simulink library "LibControllers"  (R2015b)
settings: Solver=ode45  SolverMode=SingleTasking  StartTime=0.0  StopTime=10.0  RelTol=1e-3
undefined symbols (not defined in the file or in its folder): accelCanon, adjustCoefficients, bw, depth, DiscIntNeverNeededParam, displCanon, forget, freq, initDispl, jerkCanon, kd, kdp, kf, ki, kp, maxAuthority, maxForce, nominFlow, p, R, ratedFlow, S, samplePeriod, T, velocCanon
undefined symbols (not defined in the file): fbkgen, fdp, fmax, fmin, gainRatio, interval, lagFreq, lagPhase, leadFreq, leadPhase, order, refabort, refgen, refsmooth, supplyPress, vmax, vmin
libraries: LibControllers x43, simulink x1
(part 1 of 2)
settings Model: Creator=THOENB  LastModifiedBy=Andreas
settings DataIOCC: SaveFormat=Array  SignalLoggingSaveFormat=ModelDataLogs
settings OptimizationCC: BlockReduction=off  BooleanDataType=off  ExpressionDepthLimit=2147483647
settings DebuggingCC: SaveWithParameterizedLinksMsg=none  UnderspecifiedInitializationDetection=Classic  MergeDetectMultiDrivingBlocksExec=none  SignalResolutionControl=TryResolveAllWithWarning  FcnCallInpInsideContextMsg=UseLocalSettings  StateNameClashWarn=warning  StrictBusMsg=Warning
settings HardwareCC: ProdBitPerPointer=32  ProdLargestAtomicFloat=None  ProdIntDivRoundTo=Undefined  ProdEndianess=Unspecified  ProdWordSize=32  ProdHWDeviceType=32-bit Generic  TargetUnknown=on
settings GRTTargetCC: GeneratePreprocessorConditionals=Disable all  CombineOutputUpdateFcns=off  GRTInterface=on
settings ConfigComp: CovModelRefEnable=Off

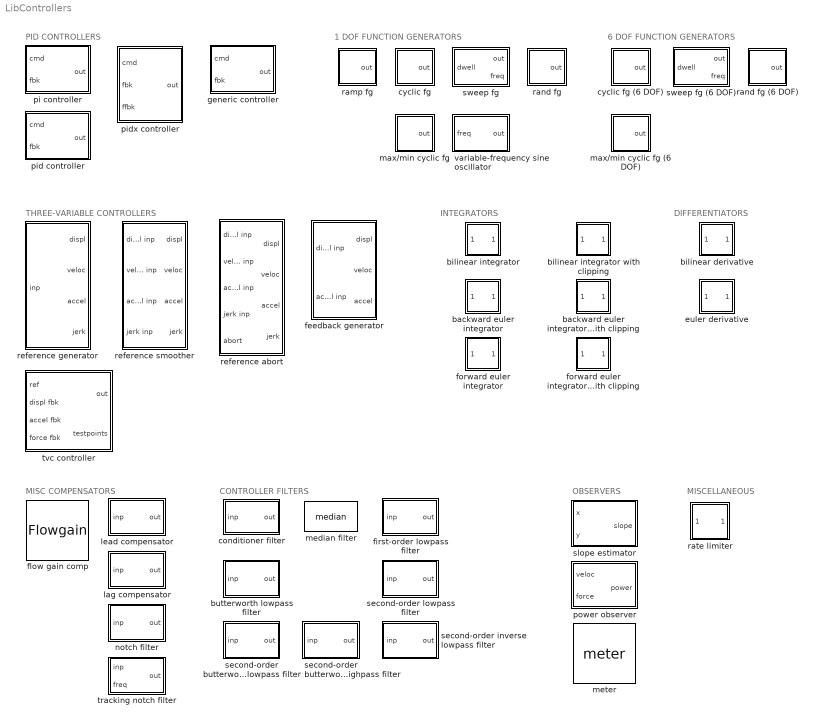
== system LibControllers ==
  note: PID CONTROLLERS
  note: MISC COMPENSATORS
  note: THREE-VARIABLE CONTROLLERS
  note: CONTROLLER FILTERS
  note: OBSERVERS
  note: 1 DOF FUNCTION GENERATORS
  note: INTEGRATORS
  note: DIFFERENTIATORS
  note: 6 DOF FUNCTION GENERATORS
  note: MISCELLANEOUS
  backward euler integrator : Subsystem  mask(Discrete Backward Euler Integrator){initialCondition=0, samplePeriod=samplePeriod}
      mask prompts: initialCondition "Initial condition"; samplePeriod "Sample period (sec)"
      mask Display: dpoly('[T]', [1 -1], 'z-')
  backward euler integrator with clipping : Subsystem  mask(Discrete Backward Euler Integrator with Clipping){initialCondition=0, maxOutput=inf, minOutput=-inf, samplePeriod=samplePeriod}
      mask prompts: initialCondition "Initial condition"; maxOutput "Maximum output"; minOutput "Minimum output"; samplePeriod "Sample period (sec)"
      mask Display: dpoly('[T]', [1 -1], 'z-')
  bilinear derivative : Subsystem  mask(Discrete Bilinear Differentiator){decay=0.9, initialCondition=0, samplePeriod=samplePeriod}
      mask prompts: decay "Decay time constant (0: backward Euler, 1: binlinear)"; initialCondition "Initial condition"; samplePeriod "Sample period"
      mask Display:
      | text(0.1,.75,'2');
      | text(0.1,.65,'_');
      | text(0.1,.25,'T');
      | text(.3,.80,'{1-z}^{-1}', 'hor','left','texmode','on');
      | text(.3,.65,'___');
      | text(.3,.30,'{1+z}^{-1}', 'hor','left','texmode','on');
  bilinear integrator : Subsystem  mask(Discrete Bilinear Integrator){initialCondition=0, samplePeriod=samplePeriod}
      mask prompts: initialCondition "Initial condition"; samplePeriod "Sample period (sec)"
      mask Display:
      | text(0.1,.75,'T');
      | text(0.1,.65,'_');
      | text(0.1,.25,'2');
      | text(.3,.80,'{1+z}^{-1}', 'hor','left','texmode','on');
      | text(.3,.65,'___');
      | text(.3,.30,'{1-z}^{-1}', 'hor','left','texmode','on');
  bilinear integrator with clipping : Subsystem  mask(Discrete Bilinear Integrator with Clipping){initialCondition=0, maxOutput=inf, minOutput=-inf, samplePeriod=samplePeriod}
      mask prompts: initialCondition "Initial condition"; maxOutput "Maximum output"; minOutput "Minimum output"; samplePeriod "Sample period (sec)"
      mask Display:
      | text(0.1,.75,'T');
      | text(0.1,.65,'_');
      | text(0.1,.25,'2');
      | text(.3,.80,'{1+z}^{-1}', 'hor','left','texmode','on');
      | text(.3,.65,'___');
      | text(.3,.30,'{1-z}^{-1}', 'hor','left','texmode','on');
  butterworth lowpass filter : Subsystem  mask(Butterworth Lowpass Filter){freq=bw, n=order, samplePeriod=samplePeriod}
      mask prompts: freq "Bandwidth (Hz)"; n "Filter order"; samplePeriod "Sample period (sec)"
      mask init:
      | fsamp = 1 / samplePeriod;
      | maxNSos	= 15;	% define maximum number of second-order sections
      | if (0 < freq) && (freq < 0.5 * fsamp) && (0 < n)
      | 	wn = freq / (0.5 * fsamp);
      | 	[z, p, k] = butter(n, wn, 'low');
      | else
      | 	[z, p, k] = tf2zpk([1], [1]);
      | end
      | [sos, g] = zp2sos(z, p, k);	% convert to second-order sections
      | 
      | % fix passband gain bug in cheby1()
      | % (note:  can't use freqz() for a single frequency)
      | wn = 0;
      | zexp = [1 exp(-1*j*wn) exp(-2*j*wn)]';
      | h = 1;
      | for i = 1:size(sos,1)
      | 	b = sos(i, 1:3);
      | 	a = sos(i, 4:6);
      | 	h = h * (b * zexp) / (a * zexp);
      | end
      | g = 1 / abs(h);
      | 
      | % check filter length
      | nSos = size(sos,1);
      | if nSos > maxNSos
      | 	fstr = ['Max number of second-order filter sections' ...
      | 			' (%u) exceeded: %u'];
      | 	error(sprintf(fstr, maxNSos, nSos));
      | end
      | 
      | % pad number of second-order filter sections up to the maximum
      | sos = [sos; repmat([1 0 0 1 0 0], maxNSos-nSos, 1)];
  conditioner filter : Subsystem  mask(Conditioner Filter){filterType=Elliptic, freq3dB=freq, samplePeriod=samplePeriod}
      mask prompts: filterType "Filter type"; freq3dB "3 dB cutoff frequency (inf, 1000, 500, 300, 100, 50 Hz)"; samplePeriod "Sample period (sec)"
      mask init:
      | fsamp = 1 / samplePeriod;
      | switch filterType
      | 	case 1	% bessel
      | 		% note:  higher 3dB frequency mapping 
      | 		% is accurate only for fsamp = 2048
      | 		if isempty(freq3dB)
      | 			freq3dB = fsamp;
      | 		elseif freq3dB == 1000
      | 			freq3dB = fsamp;
      | 		elseif freq3dB == 500
      | 			freq3dB = 1018.9;
      | 		elseif freq3dB == 300
      | 			freq3dB = 524.0;
      | 		elseif freq3dB == 100
      | 			freq3dB = 163.4;
      | 		elseif freq3dB == 50
      | 			freq3dB = 81.23;
      | 		else
      | 			freq3dB = fsamp;
      | 		end
      | 		if freq3dB > fsamp/2
      | 			a = [1];
      | 			b = [1];
      | 		else
      | 			[b, a] = besself(5, 2*pi*freq3dB);
      | 			[b, a] = bilinear(b, a, fsamp);
      | 		end
      | 	case 2	% butterworth
      | 		if freq3dB > fsamp/2
      | 			a = [1];
      | 			b = [1];
      | 		else
      | 			[b, a] = butter(5, 2*freq3dB/fsamp);
      | 		end
      | 	case 3	% elliptic
      | 		% note:  higher 3dB frequency mapping 
      | 		% is accurate only for fsamp = 2048
      | 		if isempty(freq3dB)
      | 			freq3dB = fsamp;
      | 		elseif freq3dB == 1000
      | 			freq3dB = 980.6;
      | 		elseif freq3dB == 500
      | 			freq3dB = 319.3;
      | 		elseif freq3dB == 300
      | 			freq3dB = 174.4;
      | 		elseif freq3dB == 100
      | 			freq3dB = 55.60;
      | 		elseif freq3dB == 50
      | 			freq3dB = 27.69;
      | 		else
      | 			freq3dB = fsamp;
      | 		end
      | 		if freq3dB > fsamp/2
      | 			a = [1];
      | 			b = [1];
      | 		else
      | 			[b, a] = ellip(4, 0.001, 60.0, 2*freq3dB/fsamp);
      | 		end
      | end
      mask TypeOptions filterType: Bessel | Butterworth | Elliptic
  cyclic fg : Subsystem  mask(Cyclic Function Generator){shape=Sine, ampl=1, freq=1, phase=0, spanInterval=1, samplePeriod=samplePeriod, triggered=off}
      mask prompts: ampl "Amplitude"; freq "Frequency (Hz)"; phase "Phase (deg)"; spanInterval "Span interval (sec)"; samplePeriod "Sample period (sec)"; triggered "Used in Triggered Subsystem"
      mask init:
      | if triggered
      | 	sourceSamplePeriod = -1;
      | else
      | 	sourceSamplePeriod = samplePeriod;
      | end
      | freq = max(freq, eps);
      mask TypeOptions shape: Square | Triangle | Sine
  cyclic fg (6 DOF) : Subsystem  mask(Cyclic Function Generator (6 DOF)){id=x, shape=Sine, ampl=1, freq=1, phase=0, spanInterval=1, samplePeriod=samplePeriod, dof=1:6, triggered=off}
      mask prompts: id "DOF"; ampl "Amplitude"; freq "Frequency (Hz)"; phase "Phase (deg)"; spanInterval "Span interval (sec)"; samplePeriod "Sample period (sec)"; dof "Degree-of-freedom indices (1: X; 2: Y; 3: Z; 4: Roll; 5: Pitch; 6: Yaw)"; triggered "Used in Triggered Subsystem"
      mask init:
      | if triggered
      | 	sourceSamplePeriod = -1;
      | else
      | 	sourceSamplePeriod = samplePeriod;
      | end
      mask TypeOptions id: x | y | z | roll | pitch | yaw
      mask TypeOptions shape: Square | Triangle | Sine
  euler derivative : Subsystem  mask(Discrete Euler Derivative){initialCondition=0, samplePeriod=samplePeriod}
      mask prompts: initialCondition "Initial condition"; samplePeriod "Sample period (sec)"
      mask Display: dpoly([1 -1], '[T]', 'z-')
  feedback generator : Subsystem  mask(Feedback Generator){freq=fbkgen.freq, damp=fbkgen.damp, direct=fbkgen.direct, displCanon=displCanon, velocCanon=velocCanon, accelCanon=accelCanon, initDispl=initDispl, samplePeriod=samplePeriod}
      mask prompts: freq "Crossover frequency (Hz)"; damp "Damping ratio"; direct "Direct displacement (0: indirect, 1: direct)"; displCanon "Canonical displacement units"; velocCanon "Canonical velocity units"; accelCanon "Canonical acceleration units"; initDispl "Initial displacement"; samplePeriod "Sample period (sec)"
      mask init:
      | omega = 2 * pi * freq;
      | a0    = omega * omega * omega;
      | a1    = (2 * damp + 1) * omega * omega;
      | a2    = (2 * damp + 1) * omega;
  first-order lowpass filter : Subsystem  mask(First-Order Lowpass Filter){freq=100, samplePeriod=samplePeriod}
      mask prompts: freq "Frequency (Hz)"; samplePeriod "Sample period (sec)"
      mask init:
      | fsamp = 1 / samplePeriod;
      | if ((0 < freq) && (freq < 0.5 * fsamp))
      | 	bwt	= freq * samplePeriod;
      | 	c	= 1.0 / tan(pi * bwt);	% prewarp
      | 	bwt	= 1.0 / (pi * c);
      | 	a0	= 1.0;
      | 	a1	= -exp(-2 * pi * bwt);
      | 	b0	= 1 + a1;
      | 	b1	= 0;
      | 	a	= [a0 a1];
      | 	b	= [b0 b1];
      | else
      | 	a = [1];
      | 	b = [1];
      | end
  flow gain comp : S-Function  FunctionName=Flowgain  Parameters=[satAuth droopAuth switchAuth ratedFlow nominFlow nomPress minPress maxForce]  SFunctionDeploymentMode=off  EnableBusSupport=off  mask(Flow Gain Compensator){satAuth=1, droopAuth=1, switchAuth=1, ratedFlow=ratedFlow, nominFlow=nominFlow, nomPress=supplyPress, minPress=supplyPress/3, maxForce=maxForce}
      mask prompts: satAuth "Valve saturation authority"; droopAuth "Supply pressure droop authority"; switchAuth "Pressure switching authority"; ratedFlow "Rated flow"; nominFlow "Nominal flow"; nomPress "Nominal supply pressure"; minPress "Minimum supply pressure"; maxForce "Maximum force at nominal supply pressure"
      mask Display:
      | disp('');
      | port_label('input', 1, 'inp');
      | port_label('input', 2, 'press');
      | port_label('input', 3, 'force');
      | port_label('output', 1, 'out');
      | port_label('output', 2, 'gain');
  forward euler integrator : Subsystem  mask(Discrete Forward Euler Integrator){initialCondition=0, samplePeriod=samplePeriod}
      mask prompts: initialCondition "Initial condition"; samplePeriod "Sample period (sec)"
      mask Display:
      | text(.25,.80,'{Tz}^{-1}', 'hor','left','texmode','on');
      | text(.25,.65,'___');
      | text(.25,.30,'{1-z}^{-1}', 'hor','left','texmode','on');
  forward euler integrator with clipping : Subsystem  mask(Discrete Forward Euler Integrator with Clipping){initialCondition=0, maxOutput=inf, minOutput=-inf, samplePeriod=samplePeriod}
      mask prompts: initialCondition "Initial condition"; maxOutput "Maximum output"; minOutput "Minimum output"; samplePeriod "Sample period (sec)"
      mask Display:
      | text(.25,.80,'{Tz}^{-1}', 'hor','left','texmode','on');
      | text(.25,.65,'___');
      | text(.25,.30,'{1-z}^{-1}', 'hor','left','texmode','on');
  generic controller : Subsystem  mask(Generic Controller){R=R, S=S, T=T, k=1}
      mask prompts: R "Regression polynomial"; S "Feedback polynomial"; T "Feedforward polynomial"; k "Output scaling"
  lag compensator : Subsystem  mask(Lag compensator){lagPhase=lagPhase, lagFreq=lagFreq, gainRatio=gainRatio, samplePeriod=samplePeriod}
      mask prompts: lagPhase "Lag phase ([]: use minimum possible) (deg)"; lagFreq "Lag frequency (Hz)"; gainRatio "Gain ratio (high frequency attenuation)"; samplePeriod "Sample period (sec)"
      mask init:
      | fsamp = 1 / samplePeriod;
      | if isempty(lagPhase)
      | 	lagPhase = 0;
      | end
      | 
      | % return wire if attenuation or lag frequency is zero
      | a = [1];
      | b = [1];
      | if ~(gainRatio > 0) || ~(lagFreq > 0)
      |     return
      | end
      | k         = 1 / gainRatio;
      | lagPhase  = -abs(lagPhase);
      |  
      | % determine compensator damping
      | centOmega = 2*pi*lagFreq;
      | phi       = (lagPhase / 2) * pi/180;
      | maxPhase  = 89.0 * pi/180;
      | phi       = min(phi, maxPhase);
      | tanphi    = tan(phi);
      | damp      = ((sqrt(k)-1))/(2*sqrt(sqrt(k))) / tanphi;
      |  
      | % design laplace domain compensator
      | zeroOmega = centOmega / sqrt(sqrt(k));
      | poleOmega = centOmega * sqrt(sqrt(k));
      | scale     = (poleOmega / zeroOmega)^2;
      | a         = [1 2*damp*poleOmega poleOmega^2];
      | b         = [1 2*damp*zeroOmega zeroOmega^2] * scale;
      |  
      | % transform to z domain using bilinear transformation with prewarping
      | if ~isempty(fsamp) && (lagPhase < 0)
      | 	omega = centOmega;
      | 	as   = a;
      | 	bs   = b;
      | 	a    = zeros(1, 3);
      | 	b    = zeros(1, 3);
      | 	c    = omega / tan(omega / (2*fsamp));
      | 	cc   = c * c;
      | 	d    = as(3) + as(2)*c + as(1)*cc;
      | 	a(1) = 1.0;
      | 	a(2) =  2.0*(as(3)-as(1)*cc)/d;
      | 	a(3) = (as(3)-as(2)*c+as(1)*cc)/d;
      | 	b(1) = (bs(3)+bs(2)*c+bs(1)*cc)/d;
      | 	b(2) =  2.0*(bs(3)-bs(1)*cc)/d;
      | 	b(3) = (bs(3)-bs(2)*c+bs(1)*cc)/d;
      | end
  lead compensator : Subsystem  mask(Lead compensator){leadPhase=leadPhase, leadFreq=leadFreq, gainRatio=gainRatio, samplePeriod=samplePeriod}
      mask prompts: leadPhase "Lead phase (deg)"; leadFreq "Lead frequency (Hz)"; gainRatio "Gain ratio ([]: use maximum possible)"; samplePeriod "Sample period (sec)"
      mask init:
      | fsamp = 1 / samplePeriod;
      | if isempty(gainRatio)
      | 	gainRatio = Inf;
      | end
      | 
      | % return wire if lead phase or lead frequency is zero
      | a = [1];
      | b = [1];
      | if ~(leadPhase > 0) || ~(leadFreq > 0)
      |     return
      | end
      | leadPhase = leadPhase * pi/180;
      | maxPhase  = 89.0 * pi/180;
      | 
      | % limit gain ratio
      | minGainRatio = 1.001;
      | maxGainRatio = 1000;
      | k            = min(max(gainRatio, minGainRatio), maxGainRatio);
      |  
      | % determine compensator damping
      | centOmega = 2*pi*leadFreq;
      | phi       = leadPhase / 2;
      | phi       = min(phi, maxPhase);
      | tanphi    = tan(phi);
      | damp      = ((sqrt(k) - 1) / (2*sqrt(sqrt(k)))) / tanphi;
      | damp      = min(damp, 1);
      | k         = (damp*tanphi + sqrt((damp*tanphi)^2 + 1))^4;
      |  
      | % design laplace domain compensator
      | zeroOmega = centOmega / sqrt(sqrt(k));
      | poleOmega = centOmega * sqrt(sqrt(k));
      | scale     = sqrt( (  (poleOmega^2-centOmega^2)^2 ...
      |                    + (2*damp*poleOmega*centOmega)^2) ...
      |                  / ( (zeroOmega^2-centOmega^2)^2 ...
      |                     + (2*damp*zeroOmega*centOmega)^2));
      | a         = [1 2*damp*poleOmega poleOmega^2];
      | b         = [1 2*damp*zeroOmega zeroOmega^2] * scale;
      |  
      | % transform to z domain using bilinear transformation with prewarping
      | if ~isempty(fsamp) && (leadPhase > 0)
      | 	omega = centOmega;
      | 	as   = a;
      | 	bs   = b;
      | 	a    = zeros(1, 3);
      | 	b    = zeros(1, 3);
      | 	c    = omega / tan(omega / (2*fsamp));
      | 	cc   = c * c;
      | 	d    = as(3) + as(2)*c + as(1)*cc;
      | 	a(1) = 1.0;
      | 	a(2) =  2.0*(as(3)-as(1)*cc)/d;
      | 	a(3) = (as(3)-as(2)*c+as(1)*cc)/d;
      | 	b(1) = (bs(3)+bs(2)*c+bs(1)*cc)/d;
      | 	b(2) =  2.0*(bs(3)-bs(1)*cc)/d;
      | 	b(3) = (bs(3)-bs(2)*c+bs(1)*cc)/d;
      | end
  max/min cyclic fg : Subsystem  mask(Max/Min Cyclic Function Generator){shape=Triangle, startLevel=0, endLevel=1, freq=1, samplePeriod=samplePeriod, triggered=off}
      mask prompts: startLevel "Starting level"; endLevel "Ending level"; freq "Frequency (Hz)"; samplePeriod "Sample period (sec)"; triggered "Used in Triggered Subsystem"
      mask init:
      | mean  = (startLevel + endLevel) / 2;
      | ampl  = (startLevel - endLevel) / 2;
      | phase = sign(ampl) * 90;
      | ampl  = abs(ampl);
      | if shape == 1	% square
      | 	phase = phase - 90;
      | end
      | if triggered
      | 	sourceSamplePeriod = -1;
      | else
      | 	sourceSamplePeriod = samplePeriod;
      | end
      | freq = max(freq, eps);
      mask TypeOptions shape: Square | Triangle | Sine
  max/min cyclic fg (6 DOF) : Subsystem  mask(Max/Min Cyclic Function Generator (6 DOF)){id=x, shape=Sine, startLevel=0, endLevel=1, freq=1, samplePeriod=samplePeriod, dof=1:6, triggered=off}
      mask prompts: id "DOF"; startLevel "Starting level"; endLevel "Ending level"; freq "Frequency (Hz)"; samplePeriod "Sample period (sec)"; dof "Degree-of-freedom indices (1: X; 2: Y; 3: Z; 4: Roll; 5: Pitch; 6: Yaw)"; triggered "Used in Triggered Subsystem"
      mask init:
      | mean  = (startLevel + endLevel) / 2;
      | ampl  = (startLevel - endLevel) / 2;
      | phase = sign(ampl) * 90;
      | ampl  = abs(ampl);
      | if shape == 1	% square
      | 	phase = phase - 90;
      | end
      | if triggered
      | 	sourceSamplePeriod = -1;
      | else
      | 	sourceSamplePeriod = samplePeriod;
      | end
      mask TypeOptions id: x | y | z | roll | pitch | yaw
      mask TypeOptions shape: Square | Triangle | Sine
  median filter : S-Function  FunctionName=median  Parameters=width  SFunctionDeploymentMode=off  EnableBusSupport=off  mask(Median filter){width=1}
      mask prompts: width "Glitch width (samples)"
  meter : S-Function  FunctionName=meter  Parameters=[mode band decay samplePeriod]  SFunctionDeploymentMode=off  EnableBusSupport=off  mask(Signal Meter){mode=max/min, band=0.1, decay=1, samplePeriod=samplePeriod}
      mask prompts: mode "Detector mode"; band "Sensitivity band (noise level if band mode, cycles if freq mode)"; decay "RMS/Mean averaging interval (sec if time mode, cycles if freq mode)"; samplePeriod "Sample period (sec)"
      mask help:
      | Performs the following metering operations on an input signal:
      |   * max/min
      |   * peak/valley
      |   * mean/rms
      mask TypeOptions mode: max/min | peak/valley (band) | peak/valley (freq) | mean/rms (time) | mean/rms (freq)
      mask Display:
      | disp('');
      | port_label('input', 1, 'inp');
      | port_label('input', 2, 'freq');
      | port_label('input', 3, 'reset');
      | switch mode
      | 	case {1 2 3}
      | 		port_label('output', 1, 'max');
      | 		port_label('output', 2, 'min');
      | 	case {4 5}
      | 		port_label('output', 1, 'mean');
      | 		port_label('output', 2, 'rms');
      | end
  notch filter : Subsystem  mask(Notch Filter){freq=freq, bw=bw, depth=depth, gain=1, samplePeriod=samplePeriod}
      mask prompts: freq "Center frequency (Hz)"; bw "3 dB bandwidth (Hz)"; depth "Notch depth"; gain "DC gain"; samplePeriod "Sample period (sec)"
      mask init:
      | if (0 < freq) & (freq * samplePeriod < 0.5)
      | 	t	 = tan(pi * bw * samplePeriod);	
      | 	k1	 = -cos(2 * pi * freq * samplePeriod);
      | 	k1	 = max(min(k1, 1), -1);
      | 	k2	 = (1.0 - t) / (1.0 + t);
      | 	k2	 = max(min(k2, 1), -1);
      | 	w0	 =  gain + 0.5 * depth;
      | 	w1	 = -0.5 * depth;
      | else
      | 	k1	 = 0.0;
      | 	k2	 = 0.0;
      | 	w0	 = gain;
      | 	w1	 = 0.0;
      | end
      | a1	= k1 * (1 + k2);
      | a2	= k2;
      | b	= [w0+w1*a2 (w0+w1)*a1 w1+w0*a2];
      | a	= [1 a1 a2];
  pi controller : Subsystem  mask(Proportional-Integral (PI) Controller){kp=kp, ki=ki, maxAuthority=maxAuthority, maxUnits=maxUnits, samplePeriod=samplePeriod}
      mask prompts: kp "Proportional gain"; ki "Integral gain"; maxAuthority "Max authority (percent)"; maxUnits "Max units"; samplePeriod "Sample period (sec)"
  pid controller : Subsystem  mask(Proportional-Integral-Derivative (PID) Controller){kp=kp, ki=ki, maxAuthority=maxAuthority, kd=kd, kf=kf, bw=bw, maxUnits=maxUnits, samplePeriod=samplePeriod}
      mask prompts: kp "Proportional gain"; ki "Integral gain"; maxAuthority "Max authority (percent)"; kd "Derivative gain"; kf "Feedforward gain"; bw "Bandwidth (Hz)"; maxUnits "Max units"; samplePeriod "Sample period (sec)"
  pidx controller : Subsystem  mask(Proportional-Integral-Derivative (PID) Controller){kp=kp, ki=ki, maxAuthority=maxAuthority, kd=kd, kf=kf, kdp=kdp, fdp=fdp, bw=bw, maxUnits=maxUnits, maxForceUnits=maxForceUnits, samplePeriod=samplePeriod}
      mask prompts: kp "Proportional gain"; ki "Integral gain"; maxAuthority "Max authority (percent)"; kd "Derivative gain"; kf "Feedforward gain"; kdp "Dynamic force gain"; fdp "Dynamic force frequency (Hz)"; bw "Bandwidth (Hz)"; maxUnits "Max units"; maxForceUnits "Max force units"; samplePeriod "Sample period (sec)"
      mask help: (with auxiliary stabilization input)
  power observer : Subsystem  mask(Normalized Power Observer){vmax=vmax, vmin=vmin, fmax=fmax, fmin=fmin}
      mask prompts: vmax "Maximum velocity"; vmin "Minimum velocity"; fmax "Maximum force"; fmin "Minimum force"
      mask help: Computes the power of a hydraulic actuator and normalizes it to a percent of fullscale capacity.
  ramp fg : Subsystem  mask(Ramp Function Generator){startLevel=0, endLevel=1, interval=interval, samplePeriod=samplePeriod}
      mask prompts: startLevel "Starting level"; endLevel "Ending level"; interval "Ramp interval (sec)"; samplePeriod "Sample period (sec)"
  rand fg : Subsystem  mask(Random Function Generator){shape=Flat, ampl=1, minFreq=0, maxFreq=50, spanInterval=1, samplePeriod=samplePeriod, seed=0, triggered=off, showFRF=off}
      mask prompts: ampl "RMS amplitude"; minFreq "Minimum frequency (Hz)"; maxFreq "Maximum frequency (Hz)"; spanInterval "Span interval (sec)"; samplePeriod "Sample period (sec)"; seed "Seed (use "randi(intmax)" to randomize)"; triggered "Used in Triggered Subsystem"; showFRF "Show filter frequency response"
      mask init:
      | % define maximum number of second-order sections
      | maxNSos	= 15;
      | 
      | % clip min and max frequencies to nyquist frequency
      | fsamp	= 1 / samplePeriod;
      | minFreq = min(minFreq, 0.5*fsamp);
      | maxFreq = min(maxFreq, 0.5*fsamp);
      | 
      | % design shaping filter
      | switch (shape)
      | 	case '1/F^2'	% 1/f^2 (two-pole lowpass)
      | 		% Note: Has unity amplitude at minFreq, then
      | 		% decreases at -40db per decade up to maxFreq.
      | 		minFreq = max(minFreq, 0.01*maxFreq);
      | 		k		= 0.1;
      | 		fpass	= k * minFreq;
      | 		alpha	= -exp(-2 * pi * fpass / fsamp);
      | 		a1		= 2 * alpha;
      | 		a2		= alpha^2;
      | 		b0		= (1/k)^2 * (1 + a1 + a2) * 0.25;
      | 		b1		= 2 * b0;
      | 		b2		= b0;
      | 		noiseBw = (minFreq / 3) * (1 - (minFreq / maxFreq)^3);
      | 	case '1/F'		% 1/f (one-pole lowpass)
      | 		% Note: Has unity amplitude at minFreq, then
      | 		% decreases at -20db per decade up to maxFreq.
      | 		minFreq = max(minFreq, 0.01*maxFreq);
      | 		k		= 0.1;
      | 		fpass	= k * minFreq;
      | 		alpha	= -exp(-2 * pi * fpass / fsamp);
      | 		a1		= alpha;
      | 		a2		= 0;
      | 		b0		= (1/k) * (1 + a1) * 0.5;
      | 		b1		= b0;
      | 		b2		= 0;
      | 		noiseBw = minFreq * (1 - (minFreq / maxFreq));
      | 	case 'Flat'		% flat
      | 		fpass	= maxFreq;
      | 		a1		= 0;
      | 		a2		= 0;
      | 		b0		= 1;
      | 		b1		= 0;
      | 		b2		= 0;
      | 		noiseBw = maxFreq - minFreq;
      | 	case 'F'		% f (single differentiator)
      | 		% Note:  A simple backward difference is a valid
      | 		% differentiator only up to about one half of nyquist.
      | 		% So we will select coefficients so that the slope,
      | 		% if extrapolated, would reach unity gain at nyquist
      | 		% (in reality, the gain will fall short of unity).
      | 		% These coefficients will be experimentally determined.
      | 		a1		= 0;
      | 		a2		= 0;
      | 		b0		= 0.33;
      | 		b1		= -b0;
      | 		b2		= 0;
      | 		noiseBw	= (4/3) * (maxFreq*(maxFreq/fsamp)^2 - minFreq*(minFreq/fsamp)^2);
      | 	case 'F^2'		% f^2 (double differentiator)
      | 		% Note:  See note above.
      | 		a1		= 0;
      | 		a2		= 0;
      | 		b0		= (0.33)^2;
      | 		b1		= -2 * b0;
      | 		b2		= b0;
      | 		noiseBw = (16/5) * (maxFreq*(maxFreq/fsamp)^4 - minFreq*(minFreq/fsamp)^4);
      | end
      | peakAmpl = ampl * sqrt(3) * sqrt(max(0.5*fsamp/noiseBw, 1));
      | peakAmpl = max(peakAmpl, eps);  % simulink noise block cannot tolerate zero ampl
      | [zSpf, pSpf, kSpf] = tf2zpk([b0 b1 b2], [1 a1 a2]);
      | [sosSpf, gSpf] = zp2sos(zSpf, pSpf, kSpf);	% convert to second-order sections
      | 
      | % design bandlimiting filter
      | fpassU	= maxFreq;
      | fstopU	= fpassU * 1.25;
      | fpassL	= min(minFreq, fpassU-0.001);
      | fstopL	= fpassL * 0.5;
      | rpass	= 0.01;
      | rstop	= 0.01;
      | rpassDB	= -20*log10(1-rpass);
      | rstopDB	= -20*log10(rstop);
      | if fpassL == 0
      | 		if fstopU < 0.5 * fsamp
      | 			ftype = 'lowpass';
      | 		else
      | 			ftype = 'allpass';
      | 		end
      | else
      | 		if fstopU < 0.5 * fsamp
      | 			ftype = 'bandpass';
      | 		else
      | 			ftype = 'highpass';
      | 		end	
      | end
      | switch ftype
      | 	case 'lowpass'
      | 			wp = 2 * fpassU / fsamp;
      | 			ws = 2 * fstopU / fsamp;
      | 			[n, wn]	= cheb1ord(wp, ws, rpassDB, rstopDB);
      | 			[zBlf, pBlf, kBlf] = cheby1(n, rpassDB, wn, 'low');
      | 	case 'highpass'
      | 			wp = 2 * fpassL / fsamp;
      | 			ws = 2 * fstopL / fsamp;
      | 			[n, wn]	= cheb1ord(wp, ws, rpassDB, rstopDB);
      | 			[zBlf, pBlf, kBlf] = cheby1(n, rpassDB, wn, 'high');
      | 	case 'bandpass'
      | 			wp = 2 * [fpassL fpassU] / fsamp;
      | 			ws = 2 * [fstopL fstopU] / fsamp;
      | 			[n, wn]	= cheb1ord(wp, ws, rpassDB, rstopDB);
      | 			[zBlf, pBlf, kBlf] = cheby1(n, rpassDB, wn);
      | 	case 'allpass'
      | 			[zBlf, pBlf, kBlf] = tf2zpk([1], [1]);
      | end
      | [sosBlf, gBlf] = zp2sos(zBlf, pBlf, kBlf);	% convert to second-order sections
      | 
      | % fix passband gain bug in cheby1()
      | % (note:  can't use freqz() for a single frequency)
      | switch ftype
      | 	case 'lowpass'
      | 			wn = 0;
      | 	case 'highpass'
      | 			wn = pi;
      | 	case 'bandpass'
      | 			wn = pi * wn(1);
      | 	case 'allpass'
      | 			wn = 0;
      | end
      | zexp = [1 exp(-1*j*wn) exp(-2*j*wn)]';
      | h = 1;
      | for i = 1:size(sosBlf,1)
      | 	b = sosBlf(i, 1:3);
      | 	a = sosBlf(i, 4:6);
      | 	h = h * (b * zexp) / (a * zexp);
      | end
      | gBlf = 1 / abs(h);
      | 
      | % combine shaping and bandlimiting filters
      | sos  = [sosSpf; sosBlf];
      | g    = gSpf * gBlf;
      | nSos = size(sos,1);
      | 
      | % plot filter frequency response
      | if showFRF
      | 	f    = linspace(0, fsamp/2, 8192);
      | 	hSpf = ones(size(f)) * gSpf;
      | 	hBlf = ones(size(f)) * gBlf;
      | 	for i = 1:size(sos,1)
      | 		b = sos(i, 1:3);
      | 		a = sos(i, 4:6);
      | 		if i == 1
      | 			hSpf = hSpf .* freqz(b, a, f, fsamp);
      | 		else
      | 			hBlf = hBlf .* freqz(b, a, f, fsamp);
      | 		end
      | 	end
      | 	hSpf = abs(hSpf);
      | 	hBlf = abs(hBlf);
      | 	hSpf = 20*log10(hSpf);
      | 	hBlf = 20*log10(hBlf);
      | 	plot(f, hSpf, f, hBlf, f, hSpf+hBlf);
      | 	legend('shaping filter', 'bandlimiting filter', 'combined filter');
      | 	ylabel('Magnitude (dB)');
      | 	xlabel('Frequency (Hz)');
      | 	title('Filter Frequency Response');
      | 	fstr = 'Random Fg filter:  %s with %u second-order filter sections';
      | 	disp(sprintf(fstr, ftype, nSos));
      | 
      | 	% look at filter in the Filter Visualization Tool
      | % 	fvtool(dfilt.df2sos(sosBlf, gBlf), 'Fs', fsamp);
      | end
      | 
      | % set source fg sample period
      | if triggered
      | 	sourceSamplePeriod = -1;
      | else
      | 	sourceSamplePeriod = samplePeriod;
      | end
      | 
      | % check filter length
      | if nSos > maxNSos
      | 	fstr = ['Random Fg:  Max number of second-order filter sections' ...
      | 			' (%u) exceeded: %u'];
      | 	error(sprintf(fstr, maxNSos, nSos));
      | end
      | 
      | % pad number of second-order filter sections up to the maximum
      | sos = [sos; repmat([1 0 0 1 0 0], maxNSos-nSos, 1)];
      mask TypeOptions shape: 1/F^2 | 1/F | Flat | F | F^2
  rand fg (6 DOF) : Subsystem  mask(Random Function Generator (6 DOF)){id=x, shape=Flat, ampl=1, minFreq=0, maxFreq=50, spanInterval=1, samplePeriod=samplePeriod, seed=0, dof=1:6, triggered=off, showFRF=off}
      mask prompts: id "DOF"; ampl "RMS amplitude"; minFreq "Minimum frequency (Hz)"; maxFreq "Maximum frequency (Hz)"; spanInterval "Span interval (sec)"; samplePeriod "Sample period (sec)"; seed "Seed (use "randi(intmax)" to randomize)"; dof "Degree-of-freedom indices (1: X; 2: Y; 3: Z; 4: Roll; 5: Pitch; 6: Yaw)"; triggered "Used in Triggered Subsystem"; showFRF "Show filter frequency response"
      mask init: same as LibControllers/rand fg
      mask TypeOptions id: x | y | z | roll | pitch | yaw
      mask TypeOptions shape: 1/F^2 | 1/F | Flat | F | F^2
  rate limiter : Subsystem  mask(Rate Limiter){rateMax=1, rateMin=-1, initOutput=0, rateCanon=1, samplePeriod=samplePeriod}
      mask prompts: rateMax "Rising slew rate"; rateMin "Falling slew rate"; initOutput "Initial output"; rateCanon "Canonical rate units"; samplePeriod "Sample period (sec)"
  reference abort : Subsystem  mask(Reference Abort){mode=refabort.mode, rate=refabort.rate, freq=refabort.freq, displCanon=displCanon, velocCanon=velocCanon, accelCanon=accelCanon, jerkCanon=jerkCanon, samplePeriod=samplePeriod}
      mask prompts: mode "Mode (0: return to zero, 1: return to trip level, 2: don't return)"; rate "Ramp rate"; freq "Ramp smoothing filter frequency (Hz)"; displCanon "Canonical displacement units"; velocCanon "Canonical velocity units"; accelCanon "Canonical acceleration units"; jerkCanon "Canonical jerk units"; samplePeriod "Sample period (sec)"
      mask init:
      | damp  = 1;
      | omega = 2 * pi * freq;
      | a0    = omega^3;
      | a1    = (2 * damp + 1) / omega;
      | a2    = a1 / omega;
  reference generator : Subsystem  mask(Reference Generator){mode=refgen.mode, freqHP=refgen.hpfFreq, freqLP=refgen.lpfFreq, displCanon=displCanon, velocCanon=velocCanon, accelCanon=accelCanon, jerkCanon=jerkCanon, samplePeriod=samplePeriod}
      mask prompts: mode "Mode (1: displ, 2: veloc, 3: accel)"; freqHP "Cut-in frequency (Hz)"; freqLP "Cutoff frequency (Hz)"; displCanon "Canonical displacement units"; velocCanon "Canonical velocity units"; accelCanon "Canonical acceleration units"; jerkCanon "Canonical jerk units"; samplePeriod "Sample period (sec)"
      mask init:
      | omegaHP	= 2 * pi * freqHP;
      | omegaLP	= 2 * pi * freqLP;
      | if mode == 1
      | 	damp = 0.707106781186547;
      | 	b  = omegaLP * omegaLP;
      | 	a0 = 0;
      | 	a1 = omegaLP * omegaLP;
      | 	a2 = 2 * damp * omegaLP;
      | 	canon = displCanon;
      | elseif mode == 2
      | 	damp = 0.707106781186547;
      | 	b  = omegaLP;
      | 	a0 = omegaHP * omegaHP * omegaLP;
      | 	a1 = (2 * damp * omegaLP + omegaHP) * omegaHP;
      | 	a2 = 2 * damp * omegaHP + omegaLP;
      | 	canon = velocCanon;
      | elseif mode == 3
      | 	damp = 0.5;
      | 	b  = 1;
      | 	a0 = omegaHP * omegaHP * omegaHP;
      | 	a1 = (2 * damp + 1) * omegaHP * omegaHP;
      | 	a2 = (2 * damp + 1) * omegaHP;
      | 	canon = accelCanon;
      | end
  reference smoother : Subsystem  mask(Reference Smoother){freq=refsmooth.freq, displCanon=displCanon, velocCanon=velocCanon, accelCanon=accelCanon, jerkCanon=jerkCanon, initDispl=initDispl}
      mask prompts: freq "Crossover frequency (Hz)"; displCanon "Canonical displacement units"; velocCanon "Canonical velocity units"; accelCanon "Canonical acceleration units"; jerkCanon "Canonical jerk units"; initDispl "Initial displacement"
      mask init:
      | omega = 2 * pi * freq;
      | k = omega;
  second-order butterworth highpass filter : Subsystem  mask(Second-order Butterworth Highpass Filter){freq=fdp, samplePeriod=samplePeriod}
      mask prompts: freq "Cut-in frequency (Hz)"; samplePeriod "Sample period (sec)"
      mask init:
      | bwt = freq * samplePeriod;
      | if (bwt <= 0) | (bwt >= 0.5)
      | 	a = [1];
      | 	b = [1];
      | else	% second-order butterworth
      | 	c = tan(pi * bwt);
      | 	d = (1 + sqrt(2) * c + c^2);
      | 	a = [1 -2*(1-c^2)/d (1-sqrt(2)*c+c^2)/d];
      | 	b = [1 -2 1] / d;
      | end
  second-order butterworth lowpass filter : Subsystem  mask(Second-order Butterworth Lowpass Filter){freq=bw, samplePeriod=samplePeriod}
      mask prompts: freq "Cutoff frequency (Hz)"; samplePeriod "Sample period (sec)"
      mask init:
      | bwt = freq * samplePeriod;
      | if (bwt > 0.5*0.95) 
      | 	a = [1];
      | 	b = [1];
      | else	% second-order butterworth 
      | 	c = 1 / tan(pi * bwt);
      | 	d = 1 + sqrt(2) * c + c^2;
      | 	a = [1 2*(1-c^2)/d (1-sqrt(2)*c+c^2)/d];
      | 	b = [1 2 1] * 0.25 * sum(a);
      | end
  second-order inverse lowpass filter : Subsystem  mask(Second-Order Inverse Lowpass Filter){freq=100, damp=0.5, samplePeriod=samplePeriod}
      mask prompts: freq "Frequency (Hz)"; damp "Damping"; samplePeriod "Sample period (sec)"
      mask init:
      | fsamp    = 1 / samplePeriod;
      | b        = [1];
      | a        = [1];
      | zeroFreq = 0.3;		% normalized spool filter zero freq
      | zeroDamp = 0.707;	% spool filter zero damping
      | if (   (0 < freq) && (freq < 0.5 * fsamp) ...
      | 	&& (0 < damp) && (damp <= 1))
      | 	% prewarp frequencies
      | 	omegaA	= (2.0 * fsamp) * tan(pi * freq / fsamp);
      | 	omegaB	= (2.0 * fsamp) * tan(pi * (zeroFreq*fsamp) / fsamp);
      | 
      | 	% s transfer function
      | 	scale	= omegaA^2 / omegaB^2;
      | 	a0s		= 1.0;
      | 	a1s		= 2.0 * damp * omegaA;
      | 	a2s		= omegaA^2;
      | 	b0s		= scale * 1.0;
      | 	b1s		= scale * 2.0 * zeroDamp * omegaB;
      | 	b2s		= scale * omegaB^2;
      | 
      | 	% z transfer function
      | 	wcent	= 1.0;
      | 	c		= 2.0 * fsamp / wcent;
      | 	d		= a2s + a1s*c + a0s*c*c;
      | 	a0z		= 1.0;
      | 	a1z		=  2.0*(a2s-a0s*c*c)/d;
      | 	a2z		= (a2s-a1s*c+a0s*c*c)/d;
      | 	b0z		= (b2s+b1s*c+b0s*c*c)/d;
      | 	b1z		=  2.0*(b2s-b0s*c*c)/d;
      | 	b2z		= (b2s-b1s*c+b0s*c*c)/d;
      | 	a		= [b0z b1z b2z] / b0z;
      | 	b		= [a0z a1z a2z] / b0z;
      | end
  second-order lowpass filter : Subsystem  mask(Second-Order Lowpass Filter){freq=100, damp=0.5, samplePeriod=samplePeriod}
      mask prompts: freq "Frequency (Hz)"; damp "Damping"; samplePeriod "Sample period (sec)"
      mask init:
      | fsamp = 1 / samplePeriod;
      | b     = [1];
      | a     = [1];
      | if (   (0 < freq) && (freq < 0.5 * fsamp) ...
      | 	&& (0 < damp) && (damp <= 1))
      | 	% prewarp cutoff frequency
      | 	omega	= (2.0 * fsamp) * tan(pi * freq / fsamp);
      | 
      | 	% s transfer function
      | 	a0s		= 1.0;
      | 	a1s		= 2.0 * damp * omega;
      | 	a2s		= omega^2;
      | 	b0s		= 0;
      | 	b1s		= 0;
      | 	b2s		= a2s;
      | 
      | 	% z transfer function
      | 	wcent	= 1.0;
      | 	c		= 2.0 * fsamp / wcent;
      | 	d		= a2s + a1s*c + a0s*c*c;
      | 	a0z		= 1.0;
      | 	a1z		=  2.0*(a2s-a0s*c*c)/d;
      | 	a2z		= (a2s-a1s*c+a0s*c*c)/d;
      | 	b0z		= (b2s+b1s*c+b0s*c*c)/d;
      | 	b1z		=  2.0*(b2s-b0s*c*c)/d;
      | 	b2z		= (b2s-b1s*c+b0s*c*c)/d;
      | 	a		= [a0z a1z a2z];
      | 	b		= [b0z b1z b2z];
      | end
  slope estimator : Subsystem  mask(Slope Estimator){forget=forget, minSlope=0, slope0=0, maxSlope=Inf, errcov0=1e06}
      mask prompts: forget "Forgetting factor (0: no memory, 1: no forgetting)"; minSlope "Minimum slope estimate"; slope0 "Initial slope estimate"; maxSlope "Maximum slope estimate"; errcov0 "Initial error covariance"
      mask help:
      | Reference:
      | Ljung, "System Identification Theory for the User", Prentice-Hall, 1987, p. 307, Eqn. 11.12.
  sweep fg : Subsystem  mask(Sine Sweep Function Generator){ampl=1, initialFreq=1, finalFreq=10, sweepType=linear, rate=1, spanInterval=1, samplePeriod=samplePeriod}
      mask prompts: ampl "Amplitude"; initialFreq "Initial frequency (Hz)"; finalFreq "Final frequency (Hz)"; sweepType "Sweep type"; rate "Sweep rate (linear: Hz/sec, log: oct/min)"; spanInterval "Span interval (sec)"; samplePeriod "Sample period (sec)"
      mask init:
      | switch sweepType
      | 	case 1		% linear
      | 		df	= rate * samplePeriod;
      | 		ddf	= 0;
      | 	case 2		% log
      | 		df	= 0;
      | 		ddf	= exp(rate/60 * samplePeriod * log(2)) - 1;
      | end
      | if initialFreq > finalFreq
      | 	df	= -df;
      | 	ddf	= -ddf;
      | end
      mask TypeOptions sweepType: linear | log
  sweep fg (6 DOF) : Subsystem  mask(Sine Sweep Function Generator (6 DOF)){id=x, ampl=1, initialFreq=1, finalFreq=10, sweepType=linear, rate=1, spanInterval=1, samplePeriod=samplePeriod, dof=1:6}
      mask prompts: id "DOF"; ampl "Amplitude"; initialFreq "Initial frequency (Hz)"; finalFreq "Final frequency (Hz)"; sweepType "Sweep type"; rate "Sweep rate (linear: Hz/sec, log: oct/min)"; spanInterval "Span interval (sec)"; samplePeriod "Sample period (sec)"; dof "Degree-of-freedom indices (1: X; 2: Y; 3: Z; 4: Roll; 5: Pitch; 6: Yaw)"
      mask TypeOptions id: x | y | z | roll | pitch | yaw
      mask TypeOptions sweepType: linear | log
  tracking notch filter : Subsystem  mask(Tracking Notch Filter){bw=0.1, depth=-1, gain=1, samplePeriod=samplePeriod}
      mask prompts: bw "Normalized 3 dB bandwidth (fraction of center freq)"; depth "Notch depth"; gain "DC gain"; samplePeriod "Sample period (sec)"
  tvc controller : Subsystem  mask(Three-Variable-Controller){p=p, samplePeriod=samplePeriod}
      mask prompts: p "Parameters"; samplePeriod "Sample period (sec)"
  variable-frequency sine oscillator : Subsystem  mask(Variable-Frequency Sine Oscillator){amplitude=1, samplePeriod=samplePeriod}
      mask prompts: samplePeriod "Sample period (sec)"

== system LibControllers/backward euler integrator ==
  inp : Inport
  Sum1 : Sum  Inputs=|++  SaturateOnIntegerOverflow=on  InputSameDT=on  OutDataTypeStr=Inherit: Same as first input
  T : Gain  Gain=samplePeriod
  Unit Delay1 : UnitDelay  InitialCondition=initialCondition  SampleTime=-1
  out : Outport
  wires:
  T/1 -> Sum1/1
  Sum1/1 -> out/1, Unit Delay1/1
  Unit Delay1/1 -> Sum1/2
  inp/1 -> T/1

== system LibControllers/backward euler integrator with clipping ==
  inp : Inport
  Saturation : Saturate  UpperLimit=maxOutput  LowerLimit=minOutput
  Sum1 : Sum  Inputs=|++  SaturateOnIntegerOverflow=on  InputSameDT=on  OutDataTypeStr=Inherit: Same as first input
  T : Gain  Gain=samplePeriod
  Unit Delay1 : UnitDelay  InitialCondition=initialCondition  SampleTime=-1
  out : Outport
  wires:
  Saturation/1 -> Unit Delay1/1, out/1
  inp/1 -> T/1
  Unit Delay1/1 -> Sum1/2
  Sum1/1 -> Saturation/1
  T/1 -> Sum1/1

== system LibControllers/bilinear derivative ==
  inp : Inport
  (1+decay)/T : Gain  Gain=(1+decay)/samplePeriod
  -decay : Gain  Gain=-decay
  Sum : Sum  Inputs=|+-  SaturateOnIntegerOverflow=on  InputSameDT=on  OutDataTypeStr=Inherit: Same as first input
  Sum1 : Sum  Inputs=|++  SaturateOnIntegerOverflow=on  InputSameDT=on  OutDataTypeStr=Inherit: Same as first input
  Unit Delay : UnitDelay  InitialCondition=initialCondition  SampleTime=-1
  Unit Delay1 : UnitDelay  SampleTime=-1
  out : Outport
  wires:
  Sum/1 -> (1+decay)/T/1
  Unit Delay1/1 -> -decay/1
  inp/1 -> Sum/1, Unit Delay/1
  Unit Delay/1 -> Sum/2
  -decay/1 -> Sum1/2
  Sum1/1 -> out/1, Unit Delay1/1
  (1+decay)/T/1 -> Sum1/1

== system LibControllers/bilinear integrator ==
  inp : Inport
  Sum : Sum  Inputs=|++  SaturateOnIntegerOverflow=on  InputSameDT=on  OutDataTypeStr=Inherit: Same as first input
  Sum1 : Sum  Inputs=|++  SaturateOnIntegerOverflow=on  InputSameDT=on  OutDataTypeStr=Inherit: Same as first input
  T/2 : Gain  Gain=samplePeriod/2
  Unit Delay : UnitDelay  SampleTime=-1
  Unit Delay1 : UnitDelay  InitialCondition=initialCondition  SampleTime=-1
  out : Outport
  wires:
  Sum/1 -> T/2/1
  inp/1 -> Unit Delay/1, Sum/1
  Unit Delay/1 -> Sum/2
  Unit Delay1/1 -> Sum1/2
  Sum1/1 -> Unit Delay1/1, out/1
  T/2/1 -> Sum1/1

== system LibControllers/bilinear integrator with clipping ==
  inp : Inport
  Saturation : Saturate  UpperLimit=maxOutput  LowerLimit=minOutput
  Sum : Sum  Inputs=|++  SaturateOnIntegerOverflow=on  InputSameDT=on  OutDataTypeStr=Inherit: Same as first input
  Sum1 : Sum  Inputs=|++  SaturateOnIntegerOverflow=on  InputSameDT=on  OutDataTypeStr=Inherit: Same as first input
  T/2 : Gain  Gain=samplePeriod/2
  Unit Delay : UnitDelay  SampleTime=-1
  Unit Delay1 : UnitDelay  InitialCondition=initialCondition  SampleTime=-1
  out : Outport
  wires:
  Saturation/1 -> out/1, Unit Delay1/1
  T/2/1 -> Sum1/1
  Sum1/1 -> Saturation/1
  Unit Delay1/1 -> Sum1/2
  Unit Delay/1 -> Sum/2
  inp/1 -> Sum/1, Unit Delay/1
  Sum/1 -> T/2/1

== system LibControllers/butterworth lowpass filter ==
  inp : Inport
  biquad group 1 : Subsystem  mask(Discrete Filter Group of Five Biquads){sos=sos(1:5,:)}
      mask prompts: sos "Second-order sections"
  biquad group 2 : Subsystem  mask(Discrete Filter Group of Five Biquads){sos=sos(6:10,:)}
      mask prompts: sos "Second-order sections"
  biquad group 3 : Subsystem  mask(Discrete Filter Group of Five Biquads){sos=sos(11:15,:)}
      mask prompts: sos "Second-order sections"
  gain : Gain  Gain=g
  out : Outport
  wires:
  gain/1 -> out/1
  biquad group 3/1(out) -> gain/1
  biquad group 2/1(out) -> biquad group 3/1(inp)
  biquad group 1/1(out) -> biquad group 2/1(inp)
  inp/1 -> biquad group 1/1(inp)

== system LibControllers/conditioner filter ==
  inp : Inport
  filter : DiscreteFilter  Numerator=b  Denominator=a
  out : Outport
  wires:
  inp/1 -> filter/1
  filter/1 -> out/1

== system LibControllers/cyclic fg ==
  Product : Product  RndMeth=Zero
  shape : Constant  Value=shape
  sine wave : Sin  Amplitude=ampl  Frequency=2 * pi * freq  Phase=phase * pi/180  SampleTime=sourceSamplePeriod
  span fg : LibControllers/ramp fg  SystemSampleTime=-1  startLevel=0  endLevel=1  interval=spanInterval  samplePeriod=samplePeriod
  square wave : Subsystem  mask(Repeating table){ampl=ampl, freq=freq, phase=phase, samplePeriod=samplePeriod}
      mask prompts: ampl "Amplitude"; freq "Frequency (Hz)"; phase "Phase (deg)"; samplePeriod "Sample period (sec)"
      mask help: Output a repeating sequence of numbers specified in a table of time-value pairs. Values of time should be monotonically increasing.
      mask init:
      | % phase must be positive
      | while phase < 0
      | 	phase = phase + 360;
      | end
      mask Help: Repeats cycle given in table. Time values should be monotonically increasing.
  triangle wave : Subsystem  mask(Repeating table){ampl=ampl, freq=freq, phase=phase, samplePeriod=samplePeriod}
      mask prompts: ampl "Amplitude"; freq "Frequency (Hz)"; phase "Phase (deg)"; samplePeriod "Sample period (sec)"
      mask help: Output a repeating sequence of numbers specified in a table of time-value pairs. Values of time should be monotonically increasing.
      mask init:
      | % phase must be positive
      | while phase < 0
      | 	phase = phase + 360;
      | end
      mask Help: Repeats cycle given in table. Time values should be monotonically increasing.
  waveform selector : MultiPortSwitch
  out : Outport
  wires:
  waveform selector/1 -> Product/1
  sine wave/1 -> waveform selector/4
  triangle wave/1(out) -> waveform selector/3
  square wave/1(out) -> waveform selector/2
  shape/1 -> waveform selector/1
  Product/1 -> out/1
  span fg/1 -> Product/2

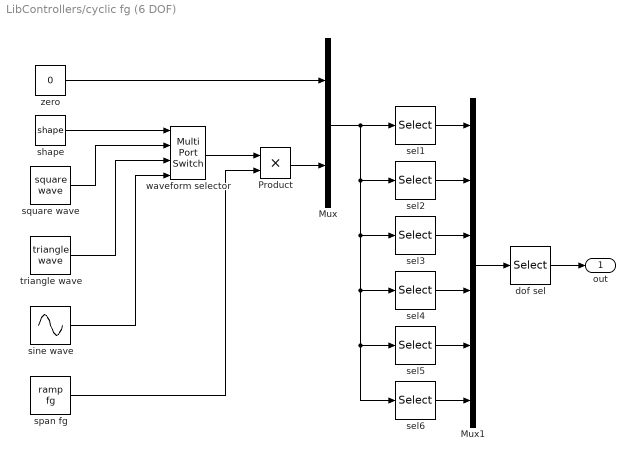
== system LibControllers/cyclic fg (6 DOF) ==
  Mux : Mux  Inputs=2
  Mux1 : Mux  Inputs=6
  Product : Product  RndMeth=Zero
  dof sel : Selector  IndexOptions=Index vector (dialog)  Indices=dof  OutputSizes=1
  sel1 : Selector  InputPortWidth=2  IndexOptions=Index vector (dialog)  Indices=(id==1)+1  OutputSizes=1
  sel2 : Selector  InputPortWidth=2  IndexOptions=Index vector (dialog)  Indices=(id==2)+1  OutputSizes=1
  sel3 : Selector  InputPortWidth=2  IndexOptions=Index vector (dialog)  Indices=(id==3)+1  OutputSizes=1
  sel4 : Selector  InputPortWidth=2  IndexOptions=Index vector (dialog)  Indices=(id==4)+1  OutputSizes=1
  sel5 : Selector  InputPortWidth=2  IndexOptions=Index vector (dialog)  Indices=(id==5)+1  OutputSizes=1
  sel6 : Selector  InputPortWidth=2  IndexOptions=Index vector (dialog)  Indices=(id==6)+1  OutputSizes=1
  shape : Constant  Value=shape
  sine wave : Sin  Amplitude=ampl  Frequency=2 * pi * freq  Phase=phase * pi/180  SampleTime=sourceSamplePeriod
  span fg : LibControllers/ramp fg  SystemSampleTime=-1  startLevel=0  endLevel=1  interval=spanInterval  samplePeriod=samplePeriod
  square wave : LibControllers/cyclic fg/square wave  SystemSampleTime=-1  ampl=ampl  freq=freq  phase=phase  samplePeriod=samplePeriod
  triangle wave : LibControllers/cyclic fg/triangle wave  SystemSampleTime=-1  ampl=ampl  freq=freq  phase=phase  samplePeriod=samplePeriod
  waveform selector : MultiPortSwitch
  zero : Constant  Value=0
  out : Outport
  wires:
  zero/1 -> Mux/1
  sel1/1 -> Mux1/1
  sel2/1 -> Mux1/2
  sel3/1 -> Mux1/3
  sel4/1 -> Mux1/4
  sel5/1 -> Mux1/5
  sel6/1 -> Mux1/6
  Mux/1 -> sel2/1, sel3/1, sel4/1, sel5/1, sel6/1, sel1/1
  sine wave/1 -> waveform selector/4
  triangle wave/1 -> waveform selector/3
  square wave/1 -> waveform selector/2
  shape/1 -> waveform selector/1
  Mux1/1 -> dof sel/1
  waveform selector/1 -> Product/1
  Product/1 -> Mux/2
  span fg/1 -> Product/2
  dof sel/1 -> out/1

== system LibControllers/euler derivative ==
  inp : Inport
  1/T : Gain  Gain=1/samplePeriod
  Sum : Sum  Inputs=|+-  SaturateOnIntegerOverflow=on  InputSameDT=on  OutDataTypeStr=Inherit: Same as first input
  Unit Delay : UnitDelay  InitialCondition=initialCondition  SampleTime=-1
  out : Outport
  wires:
  Sum/1 -> 1/T/1
  inp/1 -> Unit Delay/1, Sum/1
  Unit Delay/1 -> Sum/2
  1/T/1 -> out/1

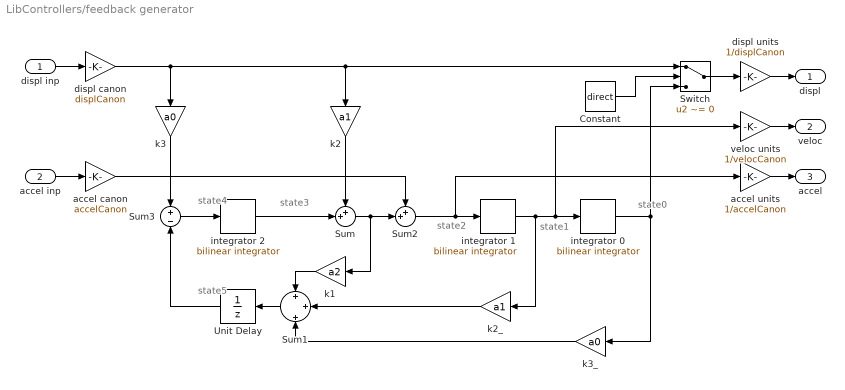
== system LibControllers/feedback generator ==
  note: state0
  note: state1
  note: state2
  note: state4
  note: state3
  note: state5
  displ inp : Inport
  accel inp : Inport  Port=2
  Constant : Constant  Value=direct
  Sum : Sum  Inputs=++|
  Sum1 : Sum  Inputs=+|+|+
  Sum2 : Sum  Inputs=++|
  Sum3 : Sum  Inputs=+|-
  Switch : Switch  Criteria=u2 ~= 0  ZeroCross=off
  Unit Delay : UnitDelay  SampleTime=-1
  accel canon : Gain  Gain=accelCanon
  accel units : Gain  Gain=1/accelCanon
  displ canon : Gain  Gain=displCanon
  displ units : Gain  Gain=1/displCanon
  integrator 0 : LibControllers/bilinear integrator  SystemSampleTime=-1  initialCondition=initDispl*displCanon  samplePeriod=samplePeriod
  integrator 1 : LibControllers/bilinear integrator  SystemSampleTime=-1  initialCondition=0  samplePeriod=samplePeriod
  integrator 2 : LibControllers/bilinear integrator  SystemSampleTime=-1  initialCondition=-initDispl*displCanon*a1  samplePeriod=samplePeriod
  k1 : Gain  Gain=a2
  k2 : Gain  Gain=a1
  k2_ : Gain  Gain=a1
  k3 : Gain  Gain=a0
  k3_ : Gain  Gain=a0
  veloc units : Gain  Gain=1/velocCanon
  displ : Outport
  veloc : Outport  Port=2
  accel : Outport  Port=3
  wires:
  k3/1 -> Sum3/1
  Sum1/1 -> Unit Delay/1
  k3_/1 -> Sum1/3
  k2_/1 -> Sum1/2
  k1/1 -> Sum1/1
  Sum3/1 -> integrator 2/1
  integrator 0/1 -> k3_/1, Switch/3
  integrator 1/1 -> k2_/1, veloc units/1, integrator 0/1
  Sum2/1 -> accel units/1, integrator 1/1
  accel canon/1 -> Sum2/1
  Sum/1 -> k1/1, Sum2/2
  integrator 2/1 -> Sum/2
  k2/1 -> Sum/1
  accel inp/1 -> accel canon/1
  displ canon/1 -> k3/1, k2/1, Switch/1
  displ inp/1 -> displ canon/1
  accel units/1 -> accel/1
  veloc units/1 -> veloc/1
  displ units/1 -> displ/1
  Unit Delay/1 -> Sum3/2
  Switch/1 -> displ units/1
  Constant/1 -> Switch/2

== system LibControllers/first-order lowpass filter ==
  inp : Inport
  discrete filter : DiscreteFilter  Numerator=b  Denominator=a
  out : Outport
  wires:
  inp/1 -> discrete filter/1
  discrete filter/1 -> out/1

== system LibControllers/forward euler integrator ==
  inp : Inport
  Sum1 : Sum  Inputs=|++  SaturateOnIntegerOverflow=on  InputSameDT=on  OutDataTypeStr=Inherit: Same as first input
  T : Gain  Gain=samplePeriod
  Unit Delay : UnitDelay  SampleTime=-1
  Unit Delay1 : UnitDelay  InitialCondition=initialCondition  SampleTime=-1
  out : Outport
  wires:
  T/1 -> Sum1/1
  Sum1/1 -> out/1, Unit Delay1/1
  Unit Delay1/1 -> Sum1/2
  Unit Delay/1 -> T/1
  inp/1 -> Unit Delay/1
